simulink model "Outer1_tmp"  (Simulink 8.3)
settings: Solver=ode45  StartTime=0.0  StopTime=10.0  RelTol=1e-3
settings Model: Creator=scaife  LastModifiedBy=hbourbou  CovSFcnEnable=on  ExtModeAutoUpdateStatusClock=off
settings DataIOCC: SignalLoggingName=sigsOut
settings DebuggingCC: SaveWithParameterizedLinksMsg=none  SignalResolutionControl=TryResolveAllWithWarning  SolverPrmCheckMsg=none  MultiTaskDSMMsg=warning  MultiTaskCondExecSysMsg=none  FrameProcessingCompatibilityMsg=error  StateNameClashWarn=none
settings HardwareCC: TargetUnknown=on
settings SFSimCC: SimParseCustomCode=off
settings GRTTargetCC: GeneratePreprocessorConditionals=Use local settings

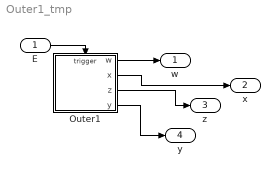
== system Outer1_tmp ==
  E : Inport
  Outer1 : Stateflow chart  TreatAsAtomicUnit=on
      settings: PermitHierarchicalResolution=ParametersOnly
  w : Outport
  x : Outport  Port=2
  z : Outport  Port=3
  y : Outport  Port=4
  wires:
  Outer1/1(w) -> w/1
  Outer1/2(x) -> x/1
  Outer1/3(z) -> z/1
  Outer1/4(y) -> y/1
  E/1 -> Outer1/Trigger

== stateflow chart Outer1 ==
  state A/
    en: z++;
    ex: w++;
  A -> A : E{x++;}/y++;
  (default) -> A
  data: w output int32; x output int32; z output int32; y output int32
  events: E input EITHER_EDGE_EVENT
